simulink model "basicElectronicCircuits"  (R2021a)
settings: Solver=VariableStepAuto  StartTime=0.0  StopTime=.1  MaxStep=10e-5  RelTol=1e-3
libraries: spsSeriesRLCBranchLib x6, spsVoltageMeasurementLib x6, spsDiodeLib x5, spsGroundLib x5, spsACVoltageSourceLib x3, spsCurrentMeasurementLib x2, spsControlledVoltageSourceLib x1, spspowerguiLib x1
settings Model: Creator=User  LastModifiedBy=User

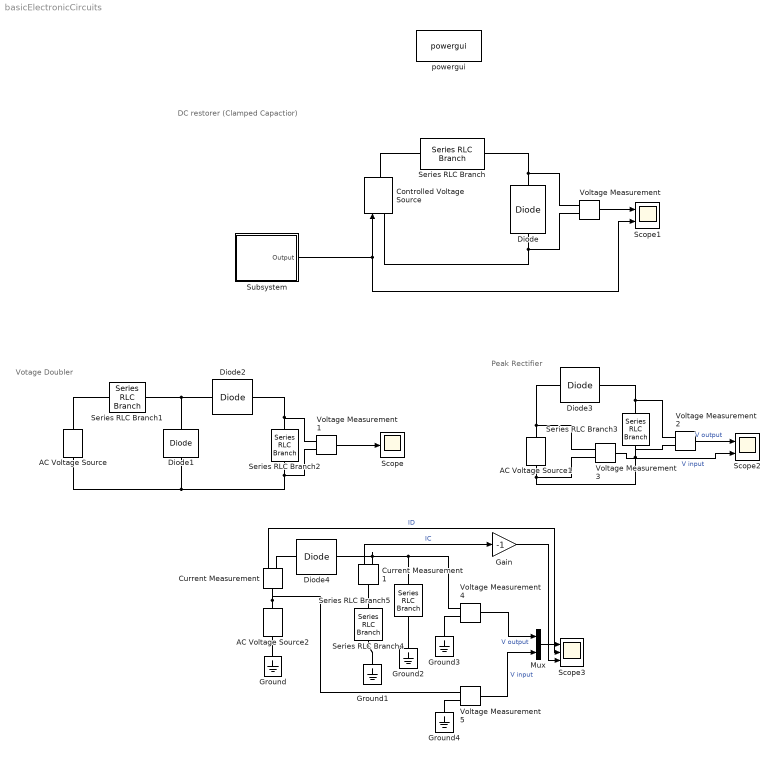
== system basicElectronicCircuits ==
  note: Peak Rectifier
  note: Votage Doubler
  note: DC restorer (Clamped Capactior)
  AC Voltage Source : spsACVoltageSourceLib/AC Voltage Source  Amplitude=100  Phase=0  Frequency=50  SampleTime=0  Measurements=None  BusType=swing  Pref=10e3  Qref=0  Qmin=-inf  Qmax=+inf
  AC Voltage Source1 : spsACVoltageSourceLib/AC Voltage Source  Amplitude=100  Phase=0  Frequency=50  SampleTime=0  Measurements=None  BusType=swing  Pref=10e3  Qref=0  Qmin=-inf  Qmax=+inf
  AC Voltage Source2 : spsACVoltageSourceLib/AC Voltage Source  Amplitude=100  Phase=0  Frequency=50  SampleTime=0  Measurements=None  BusType=swing  Pref=10e3  Qref=0  Qmin=-inf  Qmax=+inf
  Controlled Voltage Source : spsControlledVoltageSourceLib/Controlled Voltage Source  Initialize=on  Source_Type=AC  Amplitude=0  Phase=0  Frequency=0  Measurements=None
  Current Measurement : spsCurrentMeasurementLib/Current Measurement  PhasorSimulation=off  OutputType=Complex  PSBequivalent=0
  Current Measurement1 : spsCurrentMeasurementLib/Current Measurement  PhasorSimulation=off  OutputType=Complex  PSBequivalent=0
  Diode{,1..4} (5 alike) : spsDiodeLib/Diode  Ron=0.001  Lon=0  Vf=0.8  IC=0  UseSnubber=0  Rs=500  Cs=250e-9  Measurements=off
  Gain : Gain  Gain=-1
  Ground{,1..4} (5 alike) : spsGroundLib/Ground  LConnTagsString=a
  Mux : Mux  Inputs=2
  Scope : Scope
  Scope1 : Scope  NumInputPorts=2
  Scope2 : Scope  NumInputPorts=2
  Scope3 : Scope  NumInputPorts=3
  Series RLC Branch : spsSeriesRLCBranchLib/Series RLC Branch  LConnTagsString=__new0  RConnTagsString=__new0  BranchType=C  Resistance=1  Inductance=1e-3  SetiL0=off  InitialCurrent=0  Capacitance=1e-6  Setx0=off  InitialVoltage=0  Measurements=None
  Series RLC Branch1 : spsSeriesRLCBranchLib/Series RLC Branch  LConnTagsString=__new0  RConnTagsString=__new0  BranchType=C  Resistance=1  Inductance=1e-3  SetiL0=off  InitialCurrent=0  Capacitance=10e-6  Setx0=off  InitialVoltage=0  Measurements=None
  Series RLC Branch2 : spsSeriesRLCBranchLib/Series RLC Branch  LConnTagsString=__new0  RConnTagsString=__new0  BranchType=C  Resistance=1  Inductance=1e-3  SetiL0=off  InitialCurrent=0  Capacitance=10e-6  Setx0=off  InitialVoltage=0  Measurements=None
  Series RLC Branch3 : spsSeriesRLCBranchLib/Series RLC Branch  LConnTagsString=__new0  RConnTagsString=__new0  BranchType=C  Resistance=1  Inductance=1e-3  SetiL0=off  InitialCurrent=0  Capacitance=10e-6  Setx0=off  InitialVoltage=0  Measurements=None
  Series RLC Branch4 : spsSeriesRLCBranchLib/Series RLC Branch  LConnTagsString=__new0  RConnTagsString=__new0  BranchType=C  Resistance=1  Inductance=1e-3  SetiL0=off  InitialCurrent=0  Capacitance=10e-3  Setx0=off  InitialVoltage=0  Measurements=None
  Series RLC Branch5 : spsSeriesRLCBranchLib/Series RLC Branch  LConnTagsString=__new0  RConnTagsString=__new0  BranchType=R  Resistance=10  Inductance=1e-3  SetiL0=off  InitialCurrent=0  Capacitance=10e-6  Setx0=off  InitialVoltage=0  Measurements=None
  Subsystem : Subsystem
  Voltage Measurement{,1..5} (6 alike) : spsVoltageMeasurementLib/Voltage Measurement  PhasorSimulation=off  OutputType=Complex  PSBequivalent=0
  powergui : spspowerguiLib/powergui  Priority=1  SimulationMode=Continuous  SampleTime=50e-6  frequency=60  Iterations=50  frequencyindice=50  Pbase=100e6  ErrMax=1e-4  UnitsV=kV  UnitsW=MW  buscounter=0  FunctionMessages=off  echomessages=off  EnableUseOfTLC=off  CurrentSourceSwitches=off  DisableSnubberDevices=on  DisableRonSwitches=off  DisableVfSwitches=on  DisplayEquations=on  AutomaticDiscreteSolvers=off  SolverType=Tustin/Backward Euler (TBE)  Interpol=off  ExternalGateDelay=off  methode=off  Ts=100  x0status=blocks  SPID=on  SwTol=0  HookPort=off  NonlinearTolerance=1e-4  nMaxIteration=100  ContinueOnMaxIteration=off  RestoreLinks=warning  ResistiveCurrentMeasurement=off  Frange=[0:2:500]  Ylog=off  Xlog=on  ShowGrid=off  save=off  variable=ZData  structure=0  ZoomFFT=off  StartTime=0.0  cycles=1  DisplayStyle=1  fundamental=60  FreqAxis=off  MaxFrequency=1000  frequencyindicesteady=1  RmsSteady=1  display=off
  wires:
  Subsystem/1(Output) -> Scope1/2, Controlled Voltage Source/1
  Voltage Measurement/1 -> Scope1/1
  Voltage Measurement1/1 -> Scope/1
  Voltage Measurement2/1 -> Scope2/1  "V output"
  Voltage Measurement3/1 -> Scope2/2  "V input"
  Voltage Measurement5/1 -> Mux/2  "V input"
  Voltage Measurement4/1 -> Mux/1  "V output"
  Current Measurement/1 -> Scope3/2  "ID"
  Mux/1 -> Scope3/1
  Current Measurement1/1 -> Gain/1  "IC"
  Gain/1 -> Scope3/3
  connections:
  Series RLC Branch/LConn1 -- Controlled Voltage Source/RConn1
  Diode/RConn1 -- Voltage Measurement/LConn1 -- Series RLC Branch/RConn1
  Diode/LConn1 -- Controlled Voltage Source/LConn1 -- Voltage Measurement/LConn2
  Diode2/LConn1 -- Voltage Measurement1/LConn1 -- Series RLC Branch2/LConn1
  Diode1/LConn1 -- Diode2/RConn1 -- Series RLC Branch1/RConn1
  Diode1/RConn1 -- AC Voltage Source/LConn1 -- Voltage Measurement1/LConn2 -- Series RLC Branch2/RConn1
  Series RLC Branch1/LConn1 -- AC Voltage Source/RConn1
  AC Voltage Source1/RConn1 -- Diode3/LConn1 -- Voltage Measurement3/LConn1
  Series RLC Branch3/LConn1 -- Voltage Measurement2/LConn1 -- Diode3/RConn1
  AC Voltage Source1/LConn1 -- Voltage Measurement3/LConn2 -- Voltage Measurement2/LConn2 -- Series RLC Branch3/RConn1
  Current Measurement/LConn1 -- AC Voltage Source2/RConn1 -- Voltage Measurement5/LConn1
  Series RLC Branch4/LConn1 -- Current Measurement1/LConn1
  Ground/LConn1 -- AC Voltage Source2/LConn1
  Ground1/LConn1 -- Series RLC Branch4/RConn1
  Ground2/LConn1 -- Series RLC Branch5/RConn1
  Ground3/LConn1 -- Voltage Measurement4/LConn2
  Ground4/LConn1 -- Voltage Measurement5/LConn2
  Current Measurement/RConn1 -- Diode4/LConn1
  Series RLC Branch5/LConn1 -- Voltage Measurement4/LConn1 -- Diode4/RConn1 -- Current Measurement1/RConn1

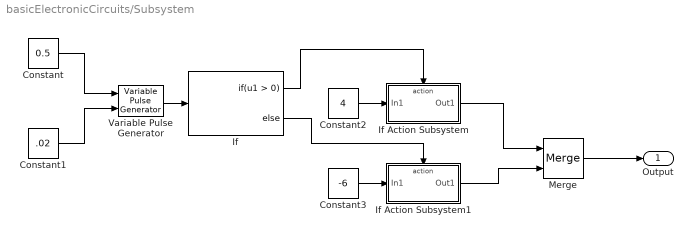
== system basicElectronicCircuits/Subsystem ==
  Constant : Constant  Value=0.5
  Constant1 : Constant  Value=.02
  Constant2 : Constant  Value=4
  Constant3 : Constant  Value=-6
  If : If
  If Action Subsystem : Subsystem  TreatAsAtomicUnit=on
  If Action Subsystem1 : Subsystem  TreatAsAtomicUnit=on
  Merge : Merge
  Variable Pulse Generator : VariablePulseGenerator  SampleTime=0.1
  Output : Outport
  wires:
  If/2 -> If Action Subsystem1/Action
  Variable Pulse Generator/1 -> If/1
  Constant3/1 -> If Action Subsystem1/1(In1)
  Constant1/1 -> Variable Pulse Generator/2
  If/1 -> If Action Subsystem/Action
  If Action Subsystem1/1(Out1) -> Merge/2
  Constant/1 -> Variable Pulse Generator/1
  Constant2/1 -> If Action Subsystem/1(In1)
  If Action Subsystem/1(Out1) -> Merge/1
  Merge/1 -> Output/1

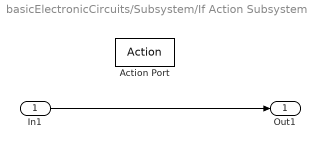
== system basicElectronicCircuits/Subsystem/If Action Subsystem ==
  In1 : Inport
  Action Port : ActionPort  ActionPortLabel=if(u1 > 0)
  Out1 : Outport
  wires:
  In1/1 -> Out1/1

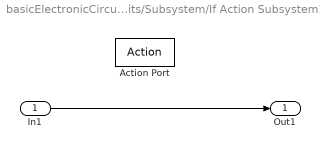
== system basicElectronicCircuits/Subsystem/If Action Subsystem1 ==
  In1 : Inport
  Action Port : ActionPort  ActionPortLabel=else
  Out1 : Outport
  wires:
  In1/1 -> Out1/1
